simulink model "WindPrototipeN"  (R2019b)
settings: Solver=ode23s  StartTime=0.0  StopTime=Ts  FixedStep=2  RelTol=5
values from neighbouring files (symbols this model uses):
  c1 = 0.51763    [matlab.mat]
  c2 = 116    [matlab.mat]
  c3 = 0.4    [matlab.mat]
  c4 = 5    [matlab.mat]
  c5 = 21    [matlab.mat]
  c6 = 0.006795    [matlab.mat]
  Tp = 2e-05    [matlab.mat]
undefined symbols (not defined in the file or in its folder): Cogent, DiscIntNeverNeededParam, Ion, Kepware, Lithium, localhost, sigbuilder_block
libraries: powerlib x266, powerlib_extras x83, simulink x30, powerlib_meascontrol x13, opclib x11, sldrtlib x8, electricdrivelib x3
(part 9 of 9)

== system WindPrototipeN/Дом 2/СОЛНЕЧНЫЕ ПАНЕЛИ1/11*2=666 V/Solar/Subsystem1/Subsystem ==
  irrad : Inport
  Controlled Current Source : powerlib/Electrical Sources/Controlled Current Source  Initialize=on  Source_Type=AC  Amplitude=0  Phase=0  Frequency=0  Measurements=None
      settings: SourceProductName=Simscape Electrical
  Diode : powerlib/Power Electronics/Diode  Ron=0.001  Lon=0  Vf=406  IC=0  UseSnubber=off  Rs=500  Cs=250e-9  Measurements=off
      settings: SourceProductName=Simscape Electrical
  Series RLC Branch : powerlib/Elements/Series RLC Branch  LConnTagsString=__new0  RConnTagsString=__new0  BranchType=R  Resistance=0.005*11  Inductance=1e-3  SetiL0=off  InitialCurrent=0  Capacitance=1e-6  Setx0=off  InitialVoltage=0  Measurements=None
      settings: SourceProductName=Simscape Electrical
  Series RLC Branch1 : powerlib/Elements/Series RLC Branch  LConnTagsString=__new0  RConnTagsString=__new0  BranchType=R  Resistance=550  Inductance=1e-3  SetiL0=off  InitialCurrent=0  Capacitance=1e-6  Setx0=off  InitialVoltage=0  Measurements=None
      settings: SourceProductName=Simscape Electrical
  + : PMIOPort  Tag=PMCPort  Side=Right
  - : PMIOPort  Tag=PMCPort  Port=2  Side=Right
  wires:
  irrad/1 -> Controlled Current Source/1
  connections:
  Controlled Current Source/LConn1 -- Diode/RConn1 -- -/RConn1 -- Series RLC Branch1/RConn1
  Diode/LConn1 -- Controlled Current Source/RConn1 -- Series RLC Branch1/LConn1 -- Series RLC Branch/LConn1
  +/RConn1 -- Series RLC Branch/RConn1

== system WindPrototipeN/Дом 2/СОЛНЕЧНЫЕ ПАНЕЛИ1/11*2=666 V/Solar/Subsystem5/Subsystem ==
  irrad : Inport
  Controlled Current Source : powerlib/Electrical Sources/Controlled Current Source  Initialize=on  Source_Type=AC  Amplitude=0  Phase=0  Frequency=0  Measurements=None
      settings: SourceProductName=Simscape Electrical
  Diode : powerlib/Power Electronics/Diode  Ron=0.001  Lon=0  Vf=406  IC=0  UseSnubber=off  Rs=500  Cs=250e-9  Measurements=off
      settings: SourceProductName=Simscape Electrical
  Series RLC Branch : powerlib/Elements/Series RLC Branch  LConnTagsString=__new0  RConnTagsString=__new0  BranchType=R  Resistance=0.005*11  Inductance=1e-3  SetiL0=off  InitialCurrent=0  Capacitance=1e-6  Setx0=off  InitialVoltage=0  Measurements=None
      settings: SourceProductName=Simscape Electrical
  Series RLC Branch1 : powerlib/Elements/Series RLC Branch  LConnTagsString=__new0  RConnTagsString=__new0  BranchType=R  Resistance=550  Inductance=1e-3  SetiL0=off  InitialCurrent=0  Capacitance=1e-6  Setx0=off  InitialVoltage=0  Measurements=None
      settings: SourceProductName=Simscape Electrical
  + : PMIOPort  Tag=PMCPort  Side=Right
  - : PMIOPort  Tag=PMCPort  Port=2  Side=Right
  wires:
  irrad/1 -> Controlled Current Source/1
  connections:
  +/RConn1 -- Series RLC Branch/RConn1
  Series RLC Branch/LConn1 -- Series RLC Branch1/LConn1 -- Controlled Current Source/RConn1 -- Diode/LConn1
  Series RLC Branch1/RConn1 -- -/RConn1 -- Diode/RConn1 -- Controlled Current Source/LConn1

== system WindPrototipeN/Дом 3/СОЛНЕЧНЫЕ ПАНЕЛИ1/11*2=666 V/Solar/Subsystem1/Subsystem ==
  irrad : Inport
  Controlled Current Source : powerlib/Electrical Sources/Controlled Current Source  Initialize=on  Source_Type=AC  Amplitude=0  Phase=0  Frequency=0  Measurements=None
      settings: SourceProductName=Simscape Electrical
  Diode : powerlib/Power Electronics/Diode  Ron=0.001  Lon=0  Vf=406  IC=0  UseSnubber=off  Rs=500  Cs=250e-9  Measurements=off
      settings: SourceProductName=Simscape Electrical
  Series RLC Branch : powerlib/Elements/Series RLC Branch  LConnTagsString=__new0  RConnTagsString=__new0  BranchType=R  Resistance=0.005*11  Inductance=1e-3  SetiL0=off  InitialCurrent=0  Capacitance=1e-6  Setx0=off  InitialVoltage=0  Measurements=None
      settings: SourceProductName=Simscape Electrical
  Series RLC Branch1 : powerlib/Elements/Series RLC Branch  LConnTagsString=__new0  RConnTagsString=__new0  BranchType=R  Resistance=550  Inductance=1e-3  SetiL0=off  InitialCurrent=0  Capacitance=1e-6  Setx0=off  InitialVoltage=0  Measurements=None
      settings: SourceProductName=Simscape Electrical
  + : PMIOPort  Tag=PMCPort  Side=Right
  - : PMIOPort  Tag=PMCPort  Port=2  Side=Right
  wires:
  irrad/1 -> Controlled Current Source/1
  connections:
  Controlled Current Source/LConn1 -- Diode/RConn1 -- -/RConn1 -- Series RLC Branch1/RConn1
  Diode/LConn1 -- Controlled Current Source/RConn1 -- Series RLC Branch1/LConn1 -- Series RLC Branch/LConn1
  +/RConn1 -- Series RLC Branch/RConn1

== system WindPrototipeN/Дом 3/СОЛНЕЧНЫЕ ПАНЕЛИ1/11*2=666 V/Solar/Subsystem5/Subsystem ==
  irrad : Inport
  Controlled Current Source : powerlib/Electrical Sources/Controlled Current Source  Initialize=on  Source_Type=AC  Amplitude=0  Phase=0  Frequency=0  Measurements=None
      settings: SourceProductName=Simscape Electrical
  Diode : powerlib/Power Electronics/Diode  Ron=0.001  Lon=0  Vf=406  IC=0  UseSnubber=off  Rs=500  Cs=250e-9  Measurements=off
      settings: SourceProductName=Simscape Electrical
  Series RLC Branch : powerlib/Elements/Series RLC Branch  LConnTagsString=__new0  RConnTagsString=__new0  BranchType=R  Resistance=0.005*11  Inductance=1e-3  SetiL0=off  InitialCurrent=0  Capacitance=1e-6  Setx0=off  InitialVoltage=0  Measurements=None
      settings: SourceProductName=Simscape Electrical
  Series RLC Branch1 : powerlib/Elements/Series RLC Branch  LConnTagsString=__new0  RConnTagsString=__new0  BranchType=R  Resistance=550  Inductance=1e-3  SetiL0=off  InitialCurrent=0  Capacitance=1e-6  Setx0=off  InitialVoltage=0  Measurements=None
      settings: SourceProductName=Simscape Electrical
  + : PMIOPort  Tag=PMCPort  Side=Right
  - : PMIOPort  Tag=PMCPort  Port=2  Side=Right
  wires:
  irrad/1 -> Controlled Current Source/1
  connections:
  +/RConn1 -- Series RLC Branch/RConn1
  Series RLC Branch/LConn1 -- Series RLC Branch1/LConn1 -- Controlled Current Source/RConn1 -- Diode/LConn1
  Series RLC Branch1/RConn1 -- -/RConn1 -- Diode/RConn1 -- Controlled Current Source/LConn1

== stateflow chart WindPrototipeN/СИСТЕМА EMS/EMS дом 2 ==
  state ESS
    Psum = WP + PV;
    Pnet = ((Psum) - Load);
    state FullSOCMode
      ConnectedLoads = 4;
      Vbatcmd = Vbatcmd_set - 10;
      Ppost = 0;
      Pin = 0;
      Pout = 0;
    state NormalOperateMode
      ConnectedLoads = 4;
      Vbatcmd = Vbatcmd_set;
      Ppost = 0;
      Pin = 0;
      Pout = 0;
    state ReadyToDistributeMode
      ConnectedLoads = 4;
      Vbatcmd = Vbatcmd_set;
      Ppost = 2;
      Pin = 0;
      Pout = 1;
    state LoadDispatcherMode
      state y = powerman(Vbat_cmd, Bpower) [function]
      state DispatchLoad3
        en: Vbatcmd = powerman(Bvol, Bp);
        ConnectedLoads = 3;
      state ReadyToRequestMode
        Vbatcmd = powerman(Bvol, Bp);
        ConnectedLoads = CurConnectLoad;
        Ppost = 1;
      state DispatchLoad2
        en: Vbatcmd = powerman(Bvol, Bp);
        ConnectedLoads = 2;
      state DispatchLoad4
        en: Vbatcmd = powerman(Bvol, Bp);
        ConnectedLoads = 1;
      state RequestMode
        en: Vbatcmd = powerman(Bvol, Bp);
        ConnectedLoads = 4;
        Pin = 1;
        Pout = 0;
      ReadyToRequestMode -> DispatchLoad3 [order 1] : [(PpostIN1 <= 1 || PpostIN2 <= 1) && after(0.25,sec)]
      DispatchLoad3 -> DispatchLoad3 [order 3] : [after(0.1,sec)]
      DispatchLoad3 -> (junction 217) [order 2] : after(0.2,sec)
      DispatchLoad3 -> DispatchLoad2 [order 1] : [SOC < 53 && after(0.25,sec)]
      DispatchLoad2 -> DispatchLoad3 [order 2] : [SOC > 53.1 && after(0.5,sec)]
      (default) -> ReadyToRequestMode
      (junction 217) -> ReadyToRequestMode : [after(0.2,sec)]
      DispatchLoad2 -> (junction 217) [order 3] : [after(0.2,sec)]
      DispatchLoad4 -> (junction 217) [order 3] : [after(0.2,sec)]
      ReadyToRequestMode -> RequestMode [order 2] : [(PpostIN1 == 2 || PpostIN2 == 2) && after(0.2, sec)]
      RequestMode -> ReadyToRequestMode [order 2] : [Pnet > 0 && after(0.25, sec)]
      DispatchLoad2 -> DispatchLoad2 [order 1] : [after(0.1,sec)]
      DispatchLoad2 -> DispatchLoad4 [order 4] : [SOC < 52 && after(0.25,sec)]
      DispatchLoad4 -> DispatchLoad2 [order 2] : [SOC > 52.5 && after(0.5,sec)]
      DispatchLoad4 -> DispatchLoad4 [order 1] : [after(0.1,sec)]
      RequestMode -> RequestMode [order 1] : [after(0.1,sec)]
    FullSOCMode -> (junction 99) [order 2] : [after(0.25, sec)]
    NormalOperateMode -> FullSOCMode [order 2] : [SOC >= 53.7 && Pnet > 0 && after(0.25,sec)]
    FullSOCMode -> NormalOperateMode [order 1] : [Pnet <= 0 && after(0.3,sec)]
    NormalOperateMode -> (junction 99) [order 1] : [Psum > k_opt*Load && after(0.1,sec)]
    (junction 99) -> ReadyToDistributeMode [order 1] : [SOC > 54.2 && [PpostIN1 == 1 || PpostIN2 == 1]]
    (junction 99) -> NormalOperateMode [order 2] : [after(0.1,sec)]
    (default) -> NormalOperateMode
    ReadyToDistributeMode -> NormalOperateMode : [(Psum < Load || SOC < 54 ||  [PpostIN1 < 1 || PpostIN2 < 1] || [PpostIN1 > 1 || PpostIN2 > 1]) && after(0.25,sec)]
    NormalOperateMode -> LoadDispatcherMode [order 3] : [SOC <= 53.2 && Pnet < 0 && after(0.2,sec)]
        | {CurConnectLoad = ConnectedLoads}
    LoadDispatcherMode -> NormalOperateMode : [SOC >= 53.4 && Pnet > 0 && after(0.1,sec)]
        | {CurConnectLoad = 4}
  state Initialization
    Vbatcmd = Vbatcmd_set;
    Ppost = 0;
    Pin = 0;
    Pout = 0;
  state ManMode
    Vbatcmd = Vbatcmd_Man;
    Pin = Pin_Man;
    Pout = Pout_Man;
    ConnectedLoads = ConnectedLoads_Man;
  (default) -> Initialization
  Initialization -> (junction 225) : [ESS == 1]
  (junction 225) -> ESS : [ESS == 1]
  ManMode -> (junction 225) : [ESS == 1]
  ESS -> ManMode : [after(0.05, sec) && ESS == 0]
  data: Vbat_cmd function_input double size=1; Bpower function_input double size=1; y function_output; Pnet local =0; WP input; PV input; Load input; Psum local =0; SOC input; Bp input; Bvol input; Vbatcmd output; Pout output; Pin output; Ppost output int8; PpostIN1 input; PpostIN2 input; ConnectedLoads output; ESS input; ConnectedLoads_Man input; Pin_Man input; Pout_Man input; Vbatcmd_Man input; CurConnectLoad local =4; Vbatcmd_set local =640; k_opt local =1.5

== stateflow chart WindPrototipeN/СИСТЕМА EMS/EMS дом 2/ESS.LoadDispatcherMode.powerman/Chart ==
  state Power_man
    (default) -> (junction 32) : {DV = (Vbatcmd - Vbatcmd_prev);
        | DP = (Bp - Bp_prev);}
    (junction 32) -> (junction 30) [order 1] : [DP*DV >= 0]
    (junction 32) -> (junction 41) [order 2] : {VoltageRef = VoltageRef - StepSize;}
    (junction 30) -> (junction 38) : {VoltageRef = VoltageRef + StepSize;}
    (junction 38) -> (junction 40) : [VoltageRef >= 640]{VoltageRef == 640;}
    (junction 41) -> (junction 40) : [VoltageRef <= 620 ]{VoltageRef == 620;}
    (junction 40) -> (junction 42) : {Vbatcmd_prev = Vbatcmd;
        | Bp_prev = Bp;}
  (default) -> Power_man : {VoltageRef = 640;}
  data: Bp input; Bp_prev local =0; DP local =0; DV local =0; VoltageRef output =640; StepSize local =2.5; Vbatcmd input; Vbatcmd_prev local =0

== stateflow chart WindPrototipeN/СИСТЕМА EMS/EMS дом 3 ==
  state ESS
    Psum = WP + PV;
    Pnet = ((Psum) - Load);
    state FullSOCMode
      ConnectedLoads = 4;
      Vbatcmd = Vbatcmd_set - 10;
      Ppost = 0;
      Pin = 0;
      Pout = 0;
    state NormalOperateMode
      ConnectedLoads = 4;
      Vbatcmd = Vbatcmd_set;
      Ppost = 0;
      Pin = 0;
      Pout = 0;
    state ReadyToDistributeMode
      ConnectedLoads = 4;
      Vbatcmd = Vbatcmd_set;
      Ppost = 2;
      Pin = 0;
      Pout = 1;
    state LoadDispatcherMode
      state y = powerman(Vbat_cmd, Bpower) [function]
      state DispatchLoad3
        en: Vbatcmd = powerman(Bvol, Bp);
        ConnectedLoads = 3;
      state ReadyToRequestMode
        Vbatcmd = powerman(Bvol, Bp);
        ConnectedLoads = CurConnectLoad;
        Ppost = 1;
      state DispatchLoad2
        en: Vbatcmd = powerman(Bvol, Bp);
        ConnectedLoads = 2;
      state DispatchLoad4
        en: Vbatcmd = powerman(Bvol, Bp);
        ConnectedLoads = 1;
      state RequestMode
        en: Vbatcmd = powerman(Bvol, Bp);
        ConnectedLoads = 4;
        Pin = 1;
        Pout = 0;
      ReadyToRequestMode -> DispatchLoad3 [order 1] : [(PpostIN1 <= 1 || PpostIN2 <= 1) && after(0.25,sec)]
      DispatchLoad3 -> DispatchLoad3 [order 3] : [after(0.1,sec)]
      DispatchLoad3 -> (junction 217) [order 2] : after(0.2,sec)
      DispatchLoad3 -> DispatchLoad2 [order 1] : [SOC < 53 && after(0.25,sec)]
      DispatchLoad2 -> DispatchLoad3 [order 2] : [SOC > 53.1 && after(0.5,sec)]
      (default) -> ReadyToRequestMode
      (junction 217) -> ReadyToRequestMode : [after(0.2,sec)]
      DispatchLoad2 -> (junction 217) [order 3] : [after(0.2,sec)]
      DispatchLoad4 -> (junction 217) [order 3] : [after(0.2,sec)]
      ReadyToRequestMode -> RequestMode [order 2] : [(PpostIN1 == 2 || PpostIN2 == 2) && after(0.2, sec)]
      RequestMode -> ReadyToRequestMode [order 2] : [Pnet > 0 && after(0.25, sec)]
      DispatchLoad2 -> DispatchLoad2 [order 1] : [after(0.1,sec)]
      DispatchLoad2 -> DispatchLoad4 [order 4] : [SOC < 52 && after(0.25,sec)]
      DispatchLoad4 -> DispatchLoad2 [order 2] : [SOC > 52.5 && after(0.5,sec)]
      DispatchLoad4 -> DispatchLoad4 [order 1] : [after(0.1,sec)]
      RequestMode -> RequestMode [order 1] : [after(0.1,sec)]
    FullSOCMode -> (junction 99) [order 2] : [after(0.25, sec)]
    NormalOperateMode -> FullSOCMode [order 2] : [SOC >= 53.7 && Pnet > 0 && after(0.25,sec)]
    FullSOCMode -> NormalOperateMode [order 1] : [Pnet <= 0 && after(0.3,sec)]
    NormalOperateMode -> (junction 99) [order 1] : [Psum > k_opt*Load && after(0.1,sec)]
    (junction 99) -> ReadyToDistributeMode [order 1] : [SOC > 54.2 && [PpostIN1 == 1 || PpostIN2 == 1]]
    (junction 99) -> NormalOperateMode [order 2] : [after(0.1,sec)]
    (default) -> NormalOperateMode
    ReadyToDistributeMode -> NormalOperateMode : [(Psum < Load || SOC < 54 ||  [PpostIN1 < 1 || PpostIN2 < 1] || [PpostIN1 > 1 || PpostIN2 > 1]) && after(0.25,sec)]
    NormalOperateMode -> LoadDispatcherMode [order 3] : [SOC <= 53.2 && Pnet < 0 && after(0.2,sec)]
        | {CurConnectLoad = ConnectedLoads}
    LoadDispatcherMode -> NormalOperateMode : [SOC >= 53.4 && Pnet > 0 && after(0.1,sec)]
        | {CurConnectLoad = 4}
  state Initialization
    Vbatcmd = Vbatcmd_set;
    Ppost = 0;
    Pin = 0;
    Pout = 0;
  state ManMode
    Vbatcmd = Vbatcmd_Man;
    Pin = Pin_Man;
    Pout = Pout_Man;
    ConnectedLoads = ConnectedLoads_Man;
  (default) -> Initialization
  Initialization -> (junction 225) : [ESS == 1]
  (junction 225) -> ESS : [ESS == 1]
  ManMode -> (junction 225) : [ESS == 1]
  ESS -> ManMode : [after(0.05, sec) && ESS == 0]
  data: Vbat_cmd function_input double size=1; Bpower function_input double size=1; y function_output; Pnet local =0; WP input; PV input; Load input; Psum local =0; SOC input; Bp input; Bvol input; Vbatcmd output; Pout output; Pin output; Ppost output int8; PpostIN1 input; PpostIN2 input; ConnectedLoads output; ESS input; ConnectedLoads_Man input; Pin_Man input; Pout_Man input; Vbatcmd_Man input; CurConnectLoad local =4; Vbatcmd_set local =640; k_opt local =1.5

== stateflow chart WindPrototipeN/СИСТЕМА EMS/EMS дом 3/ESS.LoadDispatcherMode.powerman/Chart ==
  state Power_man
    (default) -> (junction 32) : {DV = (Vbatcmd - Vbatcmd_prev);
        | DP = (Bp - Bp_prev);}
    (junction 32) -> (junction 30) [order 1] : [DP*DV >= 0]
    (junction 32) -> (junction 41) [order 2] : {VoltageRef = VoltageRef - StepSize;}
    (junction 30) -> (junction 38) : {VoltageRef = VoltageRef + StepSize;}
    (junction 38) -> (junction 40) : [VoltageRef >= 640]{VoltageRef == 640;}
    (junction 41) -> (junction 40) : [VoltageRef <= 620 ]{VoltageRef == 620;}
    (junction 40) -> (junction 42) : {Vbatcmd_prev = Vbatcmd;
        | Bp_prev = Bp;}
  (default) -> Power_man : {VoltageRef = 640;}
  data: Bp input; Bp_prev local =0; DP local =0; DV local =0; VoltageRef output =640; StepSize local =2.5; Vbatcmd input; Vbatcmd_prev local =0

== stateflow chart WindPrototipeN/СИСТЕМА EMS/Chart3 ==
  state ESS
    Psum = WP + PV;
    Pnet = ((Psum) - Load);
    state FullSOCMode
      ConnectedLoads = 4;
      Vbatcmd = Vbatcmd_set - 10;
      Ppost = 0;
      Pin = 0;
      Pout = 0;
    state NormalOperateMode
      ConnectedLoads = 4;
      Vbatcmd = Vbatcmd_set;
      Ppost = 0;
      Pin = 0;
      Pout = 0;
    state ReadyToDistributeMode
      ConnectedLoads = 4;
      Vbatcmd = Vbatcmd_set;
      Ppost = 2;
      Pin = 0;
      Pout = 1;
    state LoadDispatcherMode
      state y = powerman(Vbat_cmd, Bpower) [function]
      state DispatchLoad3
        en: Vbatcmd = powerman(Bvol, Bp);
        ConnectedLoads = 3;
      state ReadyToRequestMode
        Vbatcmd = powerman(Bvol, Bp);
        ConnectedLoads = CurConnectLoad;
        Ppost = 1;
      state DispatchLoad2
        en: Vbatcmd = powerman(Bvol, Bp);
        ConnectedLoads = 2;
      state DispatchLoad4
        en: Vbatcmd = powerman(Bvol, Bp);
        ConnectedLoads = 1;
      state RequestMode
        en: Vbatcmd = powerman(Bvol, Bp);
        ConnectedLoads = 4;
        Pin = 1;
        Pout = 0;
      ReadyToRequestMode -> DispatchLoad3 [order 1] : [(PpostIN1 <= 1 || PpostIN2 <= 1) && after(0.25,sec)]
      DispatchLoad3 -> DispatchLoad3 [order 3] : [after(0.1,sec)]
      DispatchLoad3 -> (junction 217) [order 2] : after(0.2,sec)
      DispatchLoad3 -> DispatchLoad2 [order 1] : [SOC < 53 && after(0.25,sec)]
      DispatchLoad2 -> DispatchLoad3 [order 2] : [SOC > 53.1 && after(0.5,sec)]
      (default) -> ReadyToRequestMode
      (junction 217) -> ReadyToRequestMode : [after(0.2,sec)]
      DispatchLoad2 -> (junction 217) [order 3] : [after(0.2,sec)]
      DispatchLoad4 -> (junction 217) [order 3] : [after(0.2,sec)]
      ReadyToRequestMode -> RequestMode [order 2] : [(PpostIN1 == 2 || PpostIN2 == 2) && after(0.2, sec)]
      RequestMode -> ReadyToRequestMode [order 2] : [Pnet > 0 && after(0.25, sec)]
      DispatchLoad2 -> DispatchLoad2 [order 1] : [after(0.1,sec)]
      DispatchLoad2 -> DispatchLoad4 [order 4] : [SOC < 52 && after(0.25,sec)]
      DispatchLoad4 -> DispatchLoad2 [order 2] : [SOC > 52.5 && after(0.5,sec)]
      DispatchLoad4 -> DispatchLoad4 [order 1] : [after(0.1,sec)]
      RequestMode -> RequestMode [order 1] : [after(0.1,sec)]
    FullSOCMode -> (junction 99) [order 1] : [after(0.25, sec)]
    NormalOperateMode -> FullSOCMode [order 2] : [SOC >= 53.7 && Pnet > 0 && after(0.25,sec)]
    FullSOCMode -> NormalOperateMode [order 2] : [Pnet <= 0 && after(0.3,sec)]
    NormalOperateMode -> (junction 99) [order 1] : [Psum > k_opt*Load && after(0.1,sec)]
    (junction 99) -> ReadyToDistributeMode [order 1] : [SOC > 54.2 || [PpostIN1 == 1 || PpostIN2 == 1]]
    (junction 99) -> NormalOperateMode [order 2] : [after(0.1,sec)]
    (default) -> NormalOperateMode
    ReadyToDistributeMode -> NormalOperateMode : [(Psum < Load || SOC < 54) && after(0.25,sec)]
    NormalOperateMode -> LoadDispatcherMode [order 3] : [SOC <= 53.2 && Pnet < 0 && after(0.2,sec)]
        | {CurConnectLoad = ConnectedLoads}
    LoadDispatcherMode -> NormalOperateMode : [SOC >= 53.4 && Pnet > 0 && after(0.1,sec)]
        | {CurConnectLoad = 4}
  state Initialization
    Vbatcmd = Vbatcmd_set;
    Ppost = 0;
    Pin = 0;
    Pout = 0;
  state ManMode
    Vbatcmd = Vbatcmd_Man;
    Pin = Pin_Man;
    Pout = Pout_Man;
    ConnectedLoads = ConnectedLoads_Man;
  (default) -> Initialization
  Initialization -> (junction 225) : [ESS == 1]
  (junction 225) -> ESS : [ESS == 1]
  ManMode -> (junction 225) : [ESS == 1]
  ESS -> ManMode : [after(0.05, sec) && ESS == 0]
  data: Vbat_cmd function_input double size=1; Bpower function_input double size=1; y function_output; Pnet local =0; WP input; PV input; Load input; Psum local =0; SOC input; Bp input; Bvol input; Vbatcmd output; Pout output; Pin output; Ppost output int8; PpostIN1 input; PpostIN2 input; ConnectedLoads output; ESS input; ConnectedLoads_Man input; Pin_Man input; Pout_Man input; Vbatcmd_Man input; CurConnectLoad local =4; Vbatcmd_set local =640; k_opt local =1.5

== stateflow chart WindPrototipeN/СИСТЕМА EMS/Chart3/ESS.LoadDispatcherMode.powerman/Chart ==
  state Power_man
    (default) -> (junction 32) : {DV = (Vbatcmd - Vbatcmd_prev);
        | DP = (Bp - Bp_prev);}
    (junction 32) -> (junction 30) [order 1] : [DP*DV >= 0]
    (junction 32) -> (junction 41) [order 2] : {VoltageRef = VoltageRef - StepSize;}
    (junction 30) -> (junction 38) : {VoltageRef = VoltageRef + StepSize;}
    (junction 38) -> (junction 40) : [VoltageRef >= 640]{VoltageRef == 640;}
    (junction 41) -> (junction 40) : [VoltageRef <= 620 ]{VoltageRef == 620;}
    (junction 40) -> (junction 42) : {Vbatcmd_prev = Vbatcmd;
        | Bp_prev = Bp;}
  (default) -> Power_man : {VoltageRef = 640;}
  data: Bp input; Bp_prev local =0; DP local =0; DV local =0; VoltageRef output =640; StepSize local =2.5; Vbatcmd input; Vbatcmd_prev local =0

== stateflow chart WindPrototipeN/СИСТЕМА EMS/EMS дом 1 ==
  state ESS
    Psum = WP + PV;
    Pnet = ((Psum) - Load);
    state FullSOCMode
      ConnectedLoads = 4;
      Vbatcmd = Vbatcmd_set - 10;
      Ppost = 0;
      Pin = 0;
      Pout = 0;
    state NormalOperateMode
      ConnectedLoads = 4;
      Vbatcmd = Vbatcmd_set;
      Ppost = 0;
      Pin = 0;
      Pout = 0;
    state ReadyToDistributeMode
      ConnectedLoads = 4;
      Vbatcmd = Vbatcmd_set;
      Ppost = 2;
      Pin = 0;
      Pout = 1;
    state LoadDispatcherMode
      state y = powerman(Vbat_cmd, Bpower) [function]
      state DispatchLoad3
        en: Vbatcmd = powerman(Bvol, Bp);
        ConnectedLoads = 3;
      state ReadyToRequestMode
        Vbatcmd = powerman(Bvol, Bp);
        ConnectedLoads = CurConnectLoad;
        Ppost = 1;
      state DispatchLoad2
        en: Vbatcmd = powerman(Bvol, Bp);
        ConnectedLoads = 2;
      state DispatchLoad4
        en: Vbatcmd = powerman(Bvol, Bp);
        ConnectedLoads = 1;
      state RequestMode
        en: Vbatcmd = powerman(Bvol, Bp);
        ConnectedLoads = 4;
        Pin = 1;
        Pout = 0;
      ReadyToRequestMode -> DispatchLoad3 [order 1] : [(PpostIN1 <= 1 || PpostIN2 <= 1) && after(0.25,sec)]
      DispatchLoad3 -> DispatchLoad3 [order 3] : [after(0.1,sec)]
      DispatchLoad3 -> (junction 217) [order 2] : after(0.2,sec)
      DispatchLoad3 -> DispatchLoad2 [order 1] : [SOC < 53 && after(0.25,sec)]
      DispatchLoad2 -> DispatchLoad3 [order 2] : [SOC > 53.1 && after(0.5,sec)]
      (default) -> ReadyToRequestMode
      (junction 217) -> ReadyToRequestMode : [after(0.2,sec)]
      DispatchLoad2 -> (junction 217) [order 3] : [after(0.2,sec)]
      DispatchLoad4 -> (junction 217) [order 3] : [after(0.2,sec)]
      ReadyToRequestMode -> RequestMode [order 2] : [(PpostIN1 == 2 || PpostIN2 == 2) && after(0.2, sec)]
      RequestMode -> ReadyToRequestMode [order 2] : [Pnet > 0 && after(0.25, sec)]
      DispatchLoad2 -> DispatchLoad2 [order 1] : [after(0.1,sec)]
      DispatchLoad2 -> DispatchLoad4 [order 4] : [SOC < 52 && after(0.25,sec)]
      DispatchLoad4 -> DispatchLoad2 [order 2] : [SOC > 52.5 && after(0.5,sec)]
      DispatchLoad4 -> DispatchLoad4 [order 1] : [after(0.1,sec)]
      RequestMode -> RequestMode [order 1] : [after(0.1,sec)]
    FullSOCMode -> (junction 99) [order 2] : [after(0.25, sec)]
    NormalOperateMode -> FullSOCMode [order 2] : [SOC >= 53.7 && Pnet > 0 && after(0.25,sec)]
    FullSOCMode -> NormalOperateMode [order 1] : [Pnet <= 0 && after(0.3,sec)]
    NormalOperateMode -> (junction 99) [order 1] : [Psum > k_opt*Load && after(0.1,sec)]
    (junction 99) -> ReadyToDistributeMode [order 1] : [SOC > 54.2 && [PpostIN1 == 1 || PpostIN2 == 1]]
    (junction 99) -> NormalOperateMode [order 2] : [after(0.1,sec)]
    (default) -> NormalOperateMode
    ReadyToDistributeMode -> NormalOperateMode : [(Psum < Load || SOC < 54 ||  [PpostIN1 < 1 || PpostIN2 < 1] || [PpostIN1 > 1 || PpostIN2 > 1]) && after(0.25,sec)]
    NormalOperateMode -> LoadDispatcherMode [order 3] : [SOC <= 53.2 && Pnet < 0 && after(0.2,sec)]
        | {CurConnectLoad = ConnectedLoads}
    LoadDispatcherMode -> NormalOperateMode : [SOC >= 53.4 && Pnet > 0 && after(0.1,sec)]
        | {CurConnectLoad = 4}
  state Initialization
    Vbatcmd = Vbatcmd_set;
    Ppost = 0;
    Pin = 0;
    Pout = 0;
  state ManMode
    Vbatcmd = Vbatcmd_Man;
    Pin = Pin_Man;
    Pout = Pout_Man;
    ConnectedLoads = ConnectedLoads_Man;
  (default) -> Initialization
  Initialization -> (junction 225) : [ESS == 1]
  (junction 225) -> ESS : [ESS == 1]
  ManMode -> (junction 225) : [ESS == 1]
  ESS -> ManMode : [after(0.05, sec) && ESS == 0]
  data: Vbat_cmd function_input double size=1; Bpower function_input double size=1; y function_output; Pnet local =0; WP input; PV input; Load input; Psum local =0; SOC input; Bp input; Bvol input; Vbatcmd output; Pout output; Pin output; Ppost output int8; PpostIN1 input; PpostIN2 input; ConnectedLoads output; ESS input; ConnectedLoads_Man input; Pin_Man input; Pout_Man input; Vbatcmd_Man input; CurConnectLoad local =4; Vbatcmd_set local =640; k_opt local =1.5

== stateflow chart WindPrototipeN/СИСТЕМА EMS/EMS дом 1/ESS.LoadDispatcherMode.powerman/Chart ==
  state Power_man
    (default) -> (junction 32) : {DV = (Vbatcmd - Vbatcmd_prev);
        | DP = (Bp - Bp_prev);}
    (junction 32) -> (junction 30) [order 1] : [DP*DV >= 0]
    (junction 32) -> (junction 41) [order 2] : {VoltageRef = VoltageRef - StepSize;}
    (junction 30) -> (junction 38) : {VoltageRef = VoltageRef + StepSize;}
    (junction 38) -> (junction 40) : [VoltageRef >= 640]{VoltageRef == 640;}
    (junction 41) -> (junction 40) : [VoltageRef <= 620 ]{VoltageRef == 620;}
    (junction 40) -> (junction 42) : {Vbatcmd_prev = Vbatcmd;
        | Bp_prev = Bp;}
  (default) -> Power_man : {VoltageRef = 640;}
  data: Bp input; Bp_prev local =0; DP local =0; DV local =0; VoltageRef output =640; StepSize local =2.5; Vbatcmd input; Vbatcmd_prev local =0
